simulink model "esempio_tutto"  (R2020b)
settings: Solver=VariableStepAuto  StartTime=0.0  StopTime=10.0  RelTol=1e-3
values from neighbouring files (symbols this model uses):
  b = [0,0,0]    [main_att.m]
  C_Kd = 5    [main_att.m]
  C_Kp = 5    [main_att.m]
  D = diag([0.5 1/3 0.25])    [main_att.m]
  j0 = diag([0.0109 0.0506 0.0509])    [main_att.m]
  jc = diag([0.00109 0.00109 0.00109])    [main_att.m]
  Kx = 0.012    [main_att.m]
  Ky = 0.01    [main_att.m]
  Kz = 0.008    [main_att.m]
  ng = [0.001,0.001,0.001]    [main_att.m]
  om_0 = 0.001    [main_att.m]
  R_Ka = 0.001    [main_att.m]
  R_Kd = 0.001    [main_att.m]
  R_Kl = 0.001    [main_att.m]
  R_Kn = 0.001    [main_att.m]
libraries: simulink_extras x3, vrlib x2
settings Model: Creator=jason  LastModifiedBy=jason

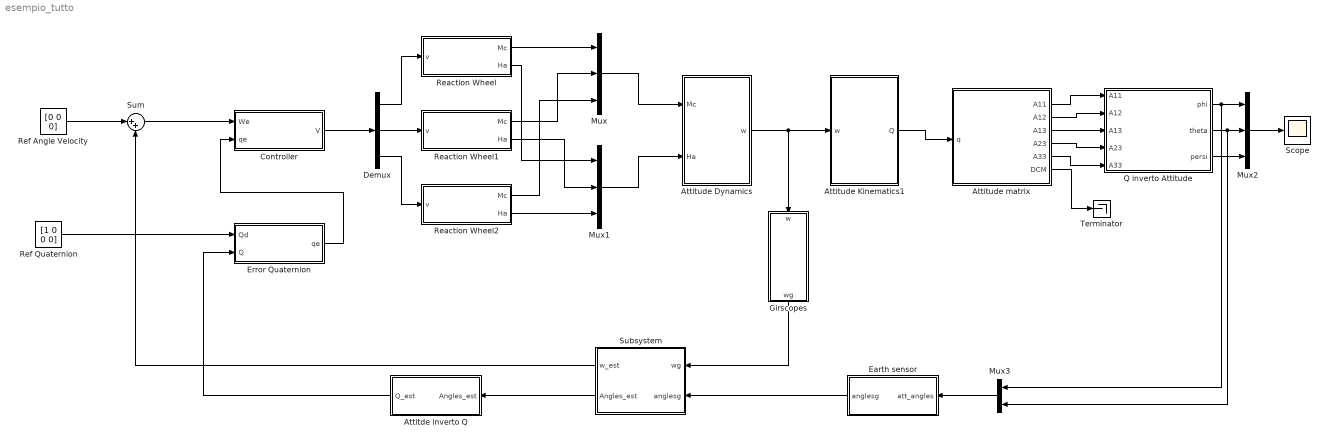
== system esempio_tutto ==
  Attitde inverto Q : Subsystem
  Attitude Dynamics : Subsystem
  Attitude Kinematics1 : Subsystem
  Attitude matrix : Subsystem
  Controller : Subsystem
  Demux : Demux  Outputs=3
  Earth sensor : Subsystem
  Error Quaternion : Subsystem
  Girscopes : Subsystem
  Mux : Mux  Inputs=3
  Mux1 : Mux  Inputs=3
  Mux2 : Mux  Inputs=3
  Mux3 : Mux  Inputs=2
  Q inverto Attitude : Subsystem
  Reaction Wheel : Subsystem
  Reaction Wheel1 : Subsystem
  Reaction Wheel2 : Subsystem
  Ref Angle Velocity : Constant  Value=[0 0 0]
  Ref Quaternion : Constant  Value=[1 0 0 0]
  Scope : Scope
  Subsystem : Subsystem
  Sum : Sum  Inputs=|++
  Terminator : Terminator
  wires:
  Sum/1 -> Controller/1(We)
  Ref Angle Velocity/1 -> Sum/1
  Error Quaternion/1(qe) -> Controller/2(qe)
  Ref Quaternion/1 -> Error Quaternion/1(Qd)
  Controller/1(V) -> Demux/1
  Demux/3 -> Reaction Wheel2/1(v)
  Demux/2 -> Reaction Wheel1/1(v)
  Demux/1 -> Reaction Wheel/1(v)
  Reaction Wheel/1(Mc) -> Mux/1
  Reaction Wheel1/1(Mc) -> Mux/2
  Reaction Wheel2/1(Mc) -> Mux/3
  Reaction Wheel/2(Ha) -> Mux1/1
  Reaction Wheel1/2(Ha) -> Mux1/2
  Reaction Wheel2/2(Ha) -> Mux1/3
  Mux/1 -> Attitude Dynamics/1(Mc)
  Mux1/1 -> Attitude Dynamics/2(Ha)
  Attitude Dynamics/1(w) -> Attitude Kinematics1/1(w), Girscopes/1(w)
  Attitude Kinematics1/1(Q) -> Attitude matrix/1(q)
  Attitude matrix/1(A11) -> Q inverto Attitude/1(A11)
  Attitude matrix/2(A12) -> Q inverto Attitude/2(A12)
  Attitude matrix/3(A13) -> Q inverto Attitude/3(A13)
  Attitude matrix/4(A23) -> Q inverto Attitude/4(A23)
  Attitude matrix/5(A33) -> Q inverto Attitude/5(A33)
  Q inverto Attitude/1(phi) -> Mux3/1, Mux2/1
  Q inverto Attitude/2(theta) -> Mux3/2, Mux2/2
  Q inverto Attitude/3(persi) -> Mux2/3
  Mux2/1 -> Scope/1
  Mux3/1 -> Earth sensor/1(att_angles)
  Girscopes/1(wg) -> Subsystem/1(wg)
  Earth sensor/1(anglesg) -> Subsystem/2(anglesg)
  Attitde inverto Q/1(Q_est) -> Error Quaternion/2(Q)
  Subsystem/2(Angles_est) -> Attitde inverto Q/1(Angles_est)
  Subsystem/1(w_est) -> Sum/2
  Attitude matrix/6(DCM) -> Terminator/1

== system esempio_tutto/Attitde inverto Q ==
  Angles_est : Inport
  MATLAB Function : MATLAB Function  TreatAsAtomicUnit=on
  Q_est : Outport
  wires:
  Angles_est/1 -> MATLAB Function/1(u)
  MATLAB Function/1(y) -> Q_est/1

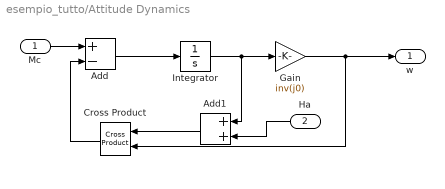
== system esempio_tutto/Attitude Dynamics ==
  Mc : Inport
  Ha : Inport  Port=2
  Add : Sum  Inputs=+-
  Add1 : Sum
  Cross Product : vrlib/Utilities/Cross Product
  Gain : Gain  Gain=inv(j0)
  Integrator : Integrator  InitialCondition=[0 0 0]
  w : Outport
  wires:
  Mc/1 -> Add/1
  Add/1 -> Integrator/1
  Integrator/1 -> Add1/1, Gain/1
  Gain/1 -> Cross Product/2, w/1
  Ha/1 -> Add1/2
  Add1/1 -> Cross Product/1
  Cross Product/1 -> Add/2

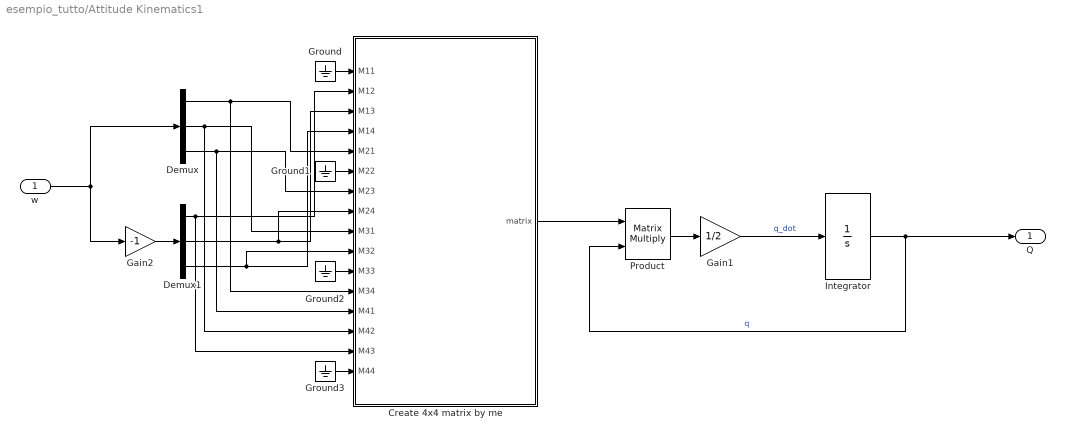
== system esempio_tutto/Attitude Kinematics1 ==
  w : Inport
  Create 4x4 matrix by me : Subsystem
  Demux : Demux  Outputs=3
  Demux1 : Demux  Outputs=3
  Gain1 : Gain  Gain=1/2
  Gain2 : Gain  Gain=-1
  Ground{,1..3} (4 alike) : Ground
  Integrator : Integrator  InitialCondition=[1 0 0 0]'
  Product : Product  Multiplication=Matrix(*)
  Q : Outport
  wires:
  Gain2/1 -> Demux1/1
  Demux/1 -> Create 4x4 matrix by me/12(M34), Create 4x4 matrix by me/5(M21)
  Demux/2 -> Create 4x4 matrix by me/14(M42), Create 4x4 matrix by me/9(M31)
  Demux/3 -> Create 4x4 matrix by me/13(M41), Create 4x4 matrix by me/7(M23)
  Demux1/1 -> Create 4x4 matrix by me/15(M43), Create 4x4 matrix by me/2(M12)
  Demux1/3 -> Create 4x4 matrix by me/10(M32), Create 4x4 matrix by me/4(M14)
  Demux1/2 -> Create 4x4 matrix by me/8(M24), Create 4x4 matrix by me/3(M13)
  Ground1/1 -> Create 4x4 matrix by me/6(M22)
  Ground/1 -> Create 4x4 matrix by me/1(M11)
  Ground2/1 -> Create 4x4 matrix by me/11(M33)
  Product/1 -> Gain1/1
  w/1 -> Demux/1, Gain2/1
  Gain1/1 -> Integrator/1  "q_dot"
  Ground3/1 -> Create 4x4 matrix by me/16(M44)
  Create 4x4 matrix by me/1(matrix) -> Product/1
  Integrator/1 -> Q/1, Product/2  "q"

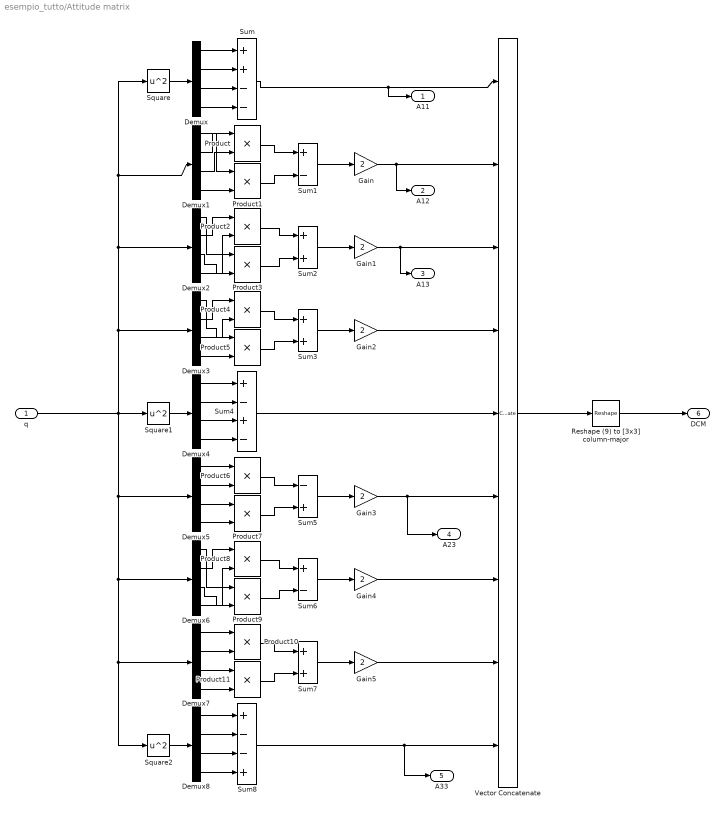
== system esempio_tutto/Attitude matrix ==
  q : Inport
  Demux{,1..8} (9 alike) : Demux
  Gain{,1..5} (6 alike) : Gain  Gain=2
  Product{,1..11} (12 alike) : Product
  Reshape (9) to [3x3] column-major : Reshape  OutputDimensionality=Customize  OutputDimensions=[3,3]
  Square : Math  Operator=square  SaturateOnIntegerOverflow=on
  Square1 : Math  Operator=square  SaturateOnIntegerOverflow=on
  Square2 : Math  Operator=square  SaturateOnIntegerOverflow=on
  Sum : Sum  Inputs=++--
  Sum1 : Sum  Inputs=+-
  Sum2 : Sum
  Sum3 : Sum
  Sum4 : Sum  Inputs=+-+-
  Sum5 : Sum  Inputs=-+
  Sum6 : Sum  Inputs=+-
  Sum7 : Sum
  Sum8 : Sum  Inputs=+--+
  Vector Concatenate : Concatenate  NumInputs=9
  A11 : Outport
  A12 : Outport  Port=2
  A13 : Outport  Port=3
  A23 : Outport  Port=4
  A33 : Outport  Port=5
  DCM : Outport  Port=6
  wires:
  Product10/1 -> Sum7/1
  Demux7/1 -> Product10/1
  Sum4/1 -> Vector Concatenate/5
  Product3/1 -> Sum2/2
  Demux5/4 -> Product7/2
  Gain5/1 -> Vector Concatenate/8
  Product11/1 -> Sum7/2
  Sum7/1 -> Gain5/1
  Gain4/1 -> Vector Concatenate/7
  Sum6/1 -> Gain4/1
  Demux5/2 -> Product6/2
  Demux7/2 -> Product10/2
  Demux5/3 -> Product7/1
  Demux5/1 -> Product6/1
  Product6/1 -> Sum5/1
  Demux3/1 -> Product5/1
  Demux6/4 -> Product8/2
  Sum3/1 -> Gain2/1
  Demux/1 -> Sum/1
  Demux6/1 -> Product9/1
  Demux4/3 -> Sum4/3
  Sum1/1 -> Gain/1
  Demux7/3 -> Product11/1
  Product7/1 -> Sum5/2
  Demux3/3 -> Product4/2
  Product4/1 -> Sum3/1
  Gain2/1 -> Vector Concatenate/4
  Demux1/3 -> Product/2
  Demux4/4 -> Sum4/4
  Demux2/2 -> Product2/1
  Product9/1 -> Sum6/2
  Demux2/1 -> Product3/1
  Demux2/4 -> Product2/2
  Demux4/2 -> Sum4/2
  Product1/1 -> Sum1/2
  Sum5/1 -> Gain3/1
  q/1 -> Square/1, Demux1/1, Demux2/1, Demux3/1, Square1/1, Demux5/1, Demux6/1, Demux7/1, Square2/1
  Product/1 -> Sum1/1
  Gain/1 -> A12/1, Vector Concatenate/2
  Product2/1 -> Sum2/1
  Sum2/1 -> Gain1/1
  Square/1 -> Demux/1
  Sum/1 -> A11/1, Vector Concatenate/1
  Demux/4 -> Sum/4
  Demux/2 -> Sum/2
  Demux3/2 -> Product4/1
  Demux6/2 -> Product8/1
  Demux/3 -> Sum/3
  Vector Concatenate/1 -> Reshape (9) to [3x3] column-major/1
  Product8/1 -> Sum6/1
  Demux8/4 -> Sum8/4
  Demux3/4 -> Product5/2
  Gain3/1 -> A23/1, Vector Concatenate/6
  Demux1/4 -> Product1/2
  Demux1/2 -> Product/1
  Demux7/4 -> Product11/2
  Demux8/2 -> Sum8/2
  Reshape (9) to [3x3] column-major/1 -> DCM/1
  Demux1/1 -> Product1/1
  Square2/1 -> Demux8/1
  Product5/1 -> Sum3/2
  Demux8/1 -> Sum8/1
  Square1/1 -> Demux4/1
  Sum8/1 -> A33/1, Vector Concatenate/9
  Gain1/1 -> A13/1, Vector Concatenate/3
  Demux4/1 -> Sum4/1
  Demux2/3 -> Product3/2
  Demux8/3 -> Sum8/3
  Demux6/3 -> Product9/2

== system esempio_tutto/Controller ==
  We : Inport
  qe : Inport  Port=2
  Gain : Gain  Gain=C_Kd  Multiplication=Matrix(K*u)
  Gain1 : Gain  Gain=C_Kp  Multiplication=Matrix(K*u)
  Quantizer : Quantizer
  Sum : Sum  Inputs=--
  V : Outport
  wires:
  We/1 -> Gain/1
  qe/1 -> Gain1/1
  Gain/1 -> Sum/1
  Gain1/1 -> Sum/2
  Sum/1 -> Quantizer/1
  Quantizer/1 -> V/1

== system esempio_tutto/Earth sensor ==
  att_angles : Inport
  Add : Sum  Inputs=+++
  Gain : Gain  Gain=b
  Quantizer : Quantizer
  Random Number : RandomNumber  Mean=0.01  SampleTime=0.1
  devi : Constant
  anglesg : Outport
  wires:
  att_angles/1 -> Add/1
  Add/1 -> Quantizer/1
  Quantizer/1 -> anglesg/1
  Random Number/1 -> Gain/1
  Gain/1 -> Add/3
  devi/1 -> Add/2

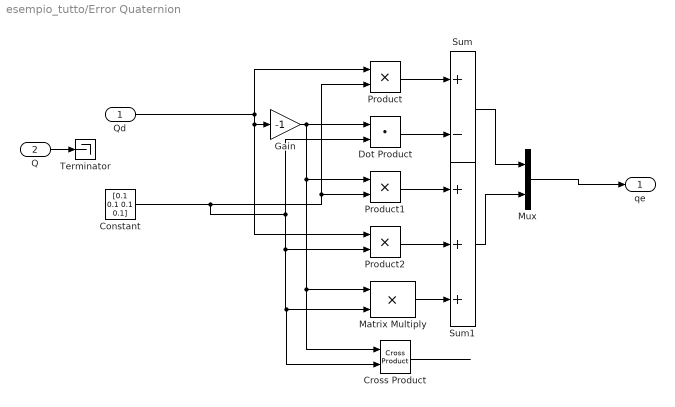
== system esempio_tutto/Error Quaternion ==
  Qd : Inport
  Q : Inport  Port=2
  Constant : Constant  Value=[0.1 0.1 0.1 0.1]
  Cross Product : vrlib/Utilities/Cross Product
  Dot Product : DotProduct  InputSameDT=on  OutDataTypeStr=Inherit: Inherit via internal rule
  Gain : Gain  Gain=-1
  Matrix Multiply : Product
  Mux : Mux  Inputs=2
  Product : Product
  Product1 : Product
  Product2 : Product
  Sum : Sum  Inputs=+-
  Sum1 : Sum  Inputs=+++
  Terminator : Terminator
  qe : Outport
  wires:
  Qd/1 -> Gain/1, Product2/1, Product/1
  Gain/1 -> Cross Product/1, Matrix Multiply/1, Product1/1, Dot Product/1
  Constant/1 -> Product/2, Product1/2, Cross Product/2, Matrix Multiply/2, Product2/2, Dot Product/2
  Product1/1 -> Sum1/1
  Product2/1 -> Sum1/2
  Matrix Multiply/1 -> Sum1/3
  Dot Product/1 -> Sum/2
  Product/1 -> Sum/1
  Sum/1 -> Mux/1
  Sum1/1 -> Mux/2
  Mux/1 -> qe/1
  Q/1 -> Terminator/1
  Cross Product/1 -> ?

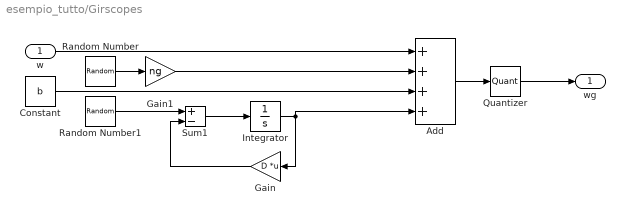
== system esempio_tutto/Girscopes ==
  w : Inport
  Add : Sum  Inputs=++++
  Constant : Constant  Value=b
  Gain : Gain  Gain=D  Multiplication=Matrix(K*u) (u vector)
  Gain1 : Gain  Gain=ng
  Integrator : Integrator  InitialCondition=nd'
  Quantizer : Quantizer
  Random Number : RandomNumber  SampleTime=0.1
  Random Number1 : RandomNumber  SampleTime=0.1
  Sum1 : Sum  Inputs=+-
  wg : Outport
  wires:
  Add/1 -> Quantizer/1
  Quantizer/1 -> wg/1
  w/1 -> Add/1
  Constant/1 -> Add/3
  Random Number/1 -> Gain1/1
  Gain1/1 -> Add/2
  Random Number1/1 -> Sum1/1
  Sum1/1 -> Integrator/1
  Integrator/1 -> Gain/1, Add/4
  Gain/1 -> Sum1/2

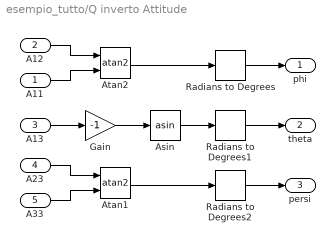
== system esempio_tutto/Q inverto Attitude ==
  A11 : Inport
  A12 : Inport  Port=2
  A13 : Inport  Port=3
  A23 : Inport  Port=4
  A33 : Inport  Port=5
  Asin : Trigonometry  Operator=asin
  Atan1 : Trigonometry  Operator=atan2
  Atan2 : Trigonometry  Operator=atan2
  Gain : Gain  Gain=-1
  Radians to Degrees : simulink_extras/Transformations/Radians to Degrees
  Radians to Degrees1 : simulink_extras/Transformations/Radians to Degrees
  Radians to Degrees2 : simulink_extras/Transformations/Radians to Degrees
  phi : Outport
  theta : Outport  Port=2
  persi : Outport  Port=3
  wires:
  A11/1 -> Atan2/2
  A12/1 -> Atan2/1
  A23/1 -> Atan1/1
  A33/1 -> Atan1/2
  A13/1 -> Gain/1
  Gain/1 -> Asin/1
  Atan2/1 -> Radians to Degrees/1
  Asin/1 -> Radians to Degrees1/1
  Atan1/1 -> Radians to Degrees2/1
  Radians to Degrees/1 -> phi/1
  Radians to Degrees1/1 -> theta/1
  Radians to Degrees2/1 -> persi/1

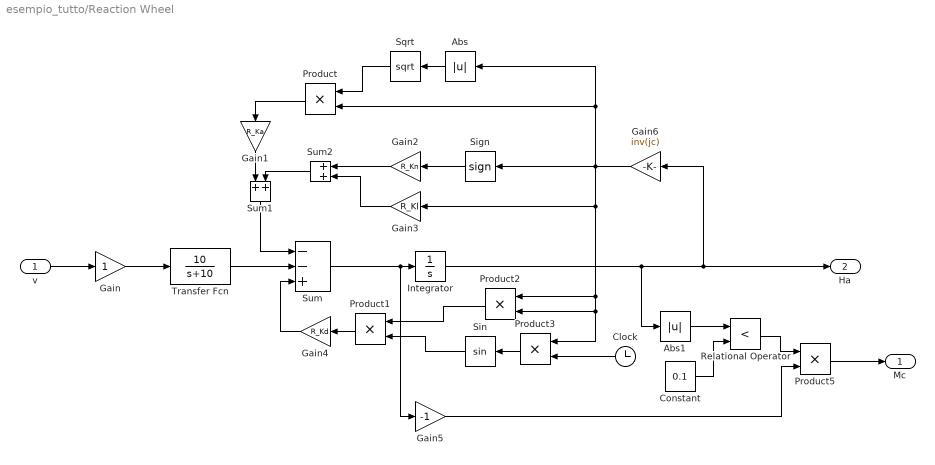
== system esempio_tutto/Reaction Wheel ==
  v : Inport
  Abs : Abs
  Abs1 : Abs
  Clock : Clock
  Constant : Constant  Value=0.1
  Gain : Gain
  Gain1 : Gain  Gain=R_Ka
  Gain2 : Gain  Gain=R_Kn
  Gain3 : Gain  Gain=R_Kl
  Gain4 : Gain  Gain=R_Kd
  Gain5 : Gain  Gain=-1
  Gain6 : Gain  Gain=inv(jc)
  Integrator : Integrator
  Product{,1..3,5} (5 alike) : Product
  Relational Operator : RelationalOperator  Operator=<  OutDataTypeStr=boolean  RndMeth=Simplest
  Sign : Signum
  Sin : Trigonometry
  Sqrt : Sqrt  SaturateOnIntegerOverflow=on
  Sum : Sum  Inputs=--+
  Sum1 : Sum
  Sum2 : Sum
  Transfer Fcn : TransferFcn  Numerator=[10]  Denominator=[1 10]
  Mc : Outport
  Ha : Outport  Port=2
  wires:
  Gain/1 -> Transfer Fcn/1
  Transfer Fcn/1 -> Sum/2
  Sum1/1 -> Sum/1
  Sum2/1 -> Sum1/2
  Gain1/1 -> Sum1/1
  Product/1 -> Gain1/1
  Abs/1 -> Sqrt/1
  Sqrt/1 -> Product/1
  Gain2/1 -> Sum2/1
  Sign/1 -> Gain2/1
  Gain3/1 -> Sum2/2
  Gain4/1 -> Sum/3
  Product1/1 -> Gain4/1
  Product3/1 -> Sin/1
  Sin/1 -> Product1/2
  Sum/1 -> Gain5/1, Integrator/1
  Integrator/1 -> Abs1/1, Ha/1, Gain6/1
  Gain6/1 -> Gain3/1, Product2/1, Product3/1, Product2/2, Product/2, Abs/1, Sign/1
  Clock/1 -> Product3/2
  Abs1/1 -> Relational Operator/1
  Constant/1 -> Relational Operator/2
  Relational Operator/1 -> Product5/1
  Gain5/1 -> Product5/2
  Product5/1 -> Mc/1
  Product2/1 -> Product1/1
  v/1 -> Gain/1

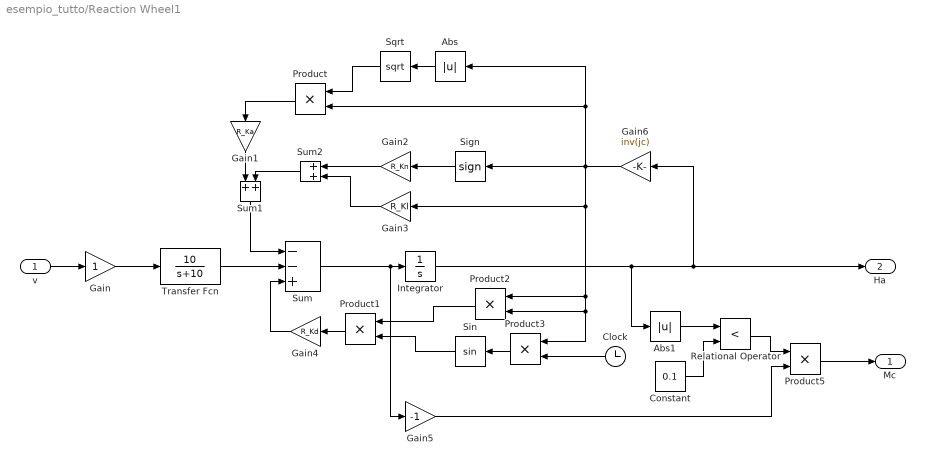
== system esempio_tutto/Reaction Wheel1 ==
  v : Inport
  Abs : Abs
  Abs1 : Abs
  Clock : Clock
  Constant : Constant  Value=0.1
  Gain : Gain
  Gain1 : Gain  Gain=R_Ka
  Gain2 : Gain  Gain=R_Kn
  Gain3 : Gain  Gain=R_Kl
  Gain4 : Gain  Gain=R_Kd
  Gain5 : Gain  Gain=-1
  Gain6 : Gain  Gain=inv(jc)
  Integrator : Integrator
  Product{,1..3,5} (5 alike) : Product
  Relational Operator : RelationalOperator  Operator=<  OutDataTypeStr=boolean  RndMeth=Simplest
  Sign : Signum
  Sin : Trigonometry
  Sqrt : Sqrt  SaturateOnIntegerOverflow=on
  Sum : Sum  Inputs=--+
  Sum1 : Sum
  Sum2 : Sum
  Transfer Fcn : TransferFcn  Numerator=[10]  Denominator=[1 10]
  Mc : Outport
  Ha : Outport  Port=2
  wires:
  Sum1/1 -> Sum/1
  Product3/1 -> Sin/1
  Relational Operator/1 -> Product5/1
  Sum/1 -> Gain5/1, Integrator/1
  Constant/1 -> Relational Operator/2
  Abs1/1 -> Relational Operator/1
  Clock/1 -> Product3/2
  Product2/1 -> Product1/1
  Transfer Fcn/1 -> Sum/2
  Product1/1 -> Gain4/1
  Gain5/1 -> Product5/2
  Gain1/1 -> Sum1/1
  Sin/1 -> Product1/2
  Integrator/1 -> Abs1/1, Ha/1, Gain6/1
  Gain3/1 -> Sum2/2
  Sum2/1 -> Sum1/2
  Product5/1 -> Mc/1
  Gain4/1 -> Sum/3
  Gain6/1 -> Gain3/1, Product2/1, Product3/1, Product2/2, Product/2, Abs/1, Sign/1
  Sign/1 -> Gain2/1
  Gain2/1 -> Sum2/1
  Sqrt/1 -> Product/1
  Product/1 -> Gain1/1
  Abs/1 -> Sqrt/1
  Gain/1 -> Transfer Fcn/1
  v/1 -> Gain/1

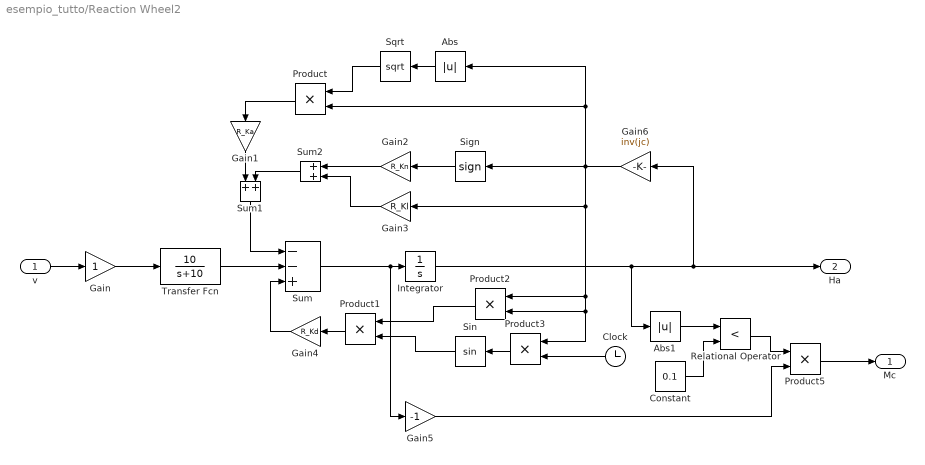
== system esempio_tutto/Reaction Wheel2 ==
  v : Inport
  Abs : Abs
  Abs1 : Abs
  Clock : Clock
  Constant : Constant  Value=0.1
  Gain : Gain
  Gain1 : Gain  Gain=R_Ka
  Gain2 : Gain  Gain=R_Kn
  Gain3 : Gain  Gain=R_Kl
  Gain4 : Gain  Gain=R_Kd
  Gain5 : Gain  Gain=-1
  Gain6 : Gain  Gain=inv(jc)
  Integrator : Integrator
  Product{,1..3,5} (5 alike) : Product
  Relational Operator : RelationalOperator  Operator=<  OutDataTypeStr=boolean  RndMeth=Simplest
  Sign : Signum
  Sin : Trigonometry
  Sqrt : Sqrt  SaturateOnIntegerOverflow=on
  Sum : Sum  Inputs=--+
  Sum1 : Sum
  Sum2 : Sum
  Transfer Fcn : TransferFcn  Numerator=[10]  Denominator=[1 10]
  Mc : Outport
  Ha : Outport  Port=2
  wires:
  Sum1/1 -> Sum/1
  Product3/1 -> Sin/1
  Relational Operator/1 -> Product5/1
  Sum/1 -> Gain5/1, Integrator/1
  Constant/1 -> Relational Operator/2
  Abs1/1 -> Relational Operator/1
  Clock/1 -> Product3/2
  Product2/1 -> Product1/1
  Transfer Fcn/1 -> Sum/2
  Product1/1 -> Gain4/1
  Gain5/1 -> Product5/2
  Gain1/1 -> Sum1/1
  Sin/1 -> Product1/2
  Integrator/1 -> Abs1/1, Ha/1, Gain6/1
  Gain3/1 -> Sum2/2
  Sum2/1 -> Sum1/2
  Product5/1 -> Mc/1
  Gain4/1 -> Sum/3
  v/1 -> Gain/1
  Gain6/1 -> Gain3/1, Product2/1, Product3/1, Product2/2, Product/2, Abs/1, Sign/1
  Sign/1 -> Gain2/1
  Gain2/1 -> Sum2/1
  Sqrt/1 -> Product/1
  Product/1 -> Gain1/1
  Abs/1 -> Sqrt/1
  Gain/1 -> Transfer Fcn/1

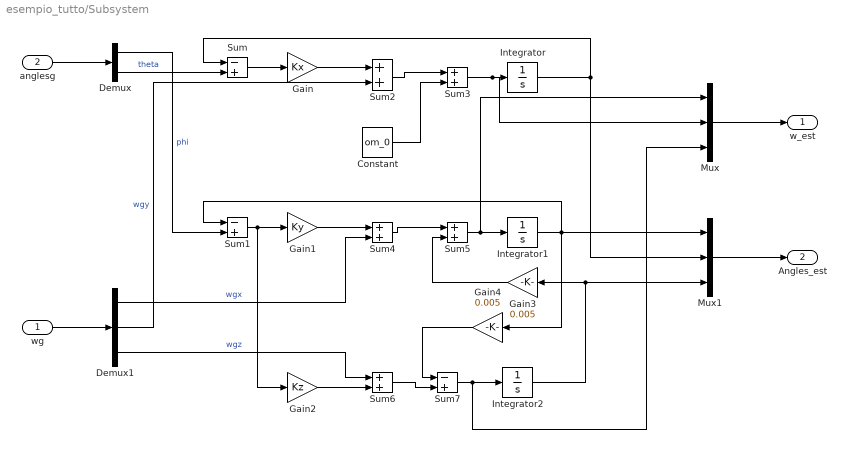
== system esempio_tutto/Subsystem ==
  wg : Inport
  anglesg : Inport  Port=2
  Constant : Constant  Value=om_0
  Demux : Demux  Outputs=2
  Demux1 : Demux  Outputs=3
  Gain : Gain  Gain=Kx
  Gain1 : Gain  Gain=Ky
  Gain2 : Gain  Gain=Kz
  Gain3 : Gain  Gain=0.005
  Gain4 : Gain  Gain=0.005
  Integrator : Integrator
  Integrator1 : Integrator
  Integrator2 : Integrator
  Mux : Mux  Inputs=3
  Mux1 : Mux  Inputs=3
  Sum : Sum  Inputs=-+
  Sum1 : Sum  Inputs=-+
  Sum{2..6} (5 alike) : Sum
  Sum7 : Sum  Inputs=-+
  w_est : Outport
  Angles_est : Outport  Port=2
  wires:
  anglesg/1 -> Demux/1
  wg/1 -> Demux1/1
  Demux/2 -> Sum/2  "theta"
  Demux/1 -> Sum1/2  "phi"
  Sum/1 -> Gain/1
  Sum1/1 -> Gain2/1, Gain1/1
  Gain/1 -> Sum2/1
  Sum2/1 -> Sum3/1
  Sum3/1 -> Mux/2, Integrator/1
  Constant/1 -> Sum3/2
  Demux1/2 -> Sum2/2  "wgy"
  Gain1/1 -> Sum4/1
  Sum4/1 -> Sum5/1
  Sum5/1 -> Integrator1/1, Mux/1
  Gain2/1 -> Sum6/2
  Sum6/1 -> Sum7/2
  Demux1/3 -> Sum6/1  "wgz"
  Demux1/1 -> Sum4/2  "wgx"
  Integrator1/1 -> Gain4/1, Mux1/1, Sum1/1
  Gain3/1 -> Sum5/2
  Sum7/1 -> Mux/3, Integrator2/1
  Gain4/1 -> Sum7/1
  Integrator2/1 -> Gain3/1, Mux1/3
  Integrator/1 -> Mux1/2, Sum/1
  Mux1/1 -> Angles_est/1
  Mux/1 -> w_est/1

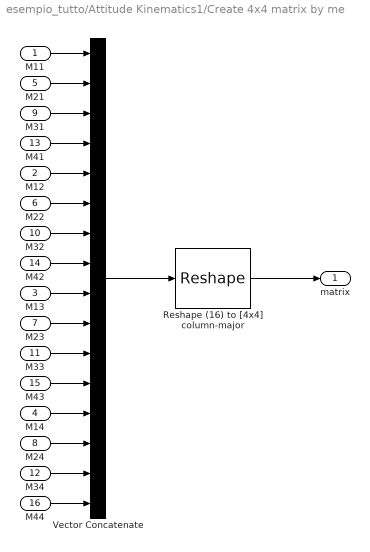
== system esempio_tutto/Attitude Kinematics1/Create 4x4 matrix by me ==
  M11 : Inport
  M12 : Inport  Port=2
  M13 : Inport  Port=3
  M14 : Inport  Port=4
  M21 : Inport  Port=5
  M22 : Inport  Port=6
  M23 : Inport  Port=7
  M24 : Inport  Port=8
  M31 : Inport  Port=9
  M32 : Inport  Port=10
  M33 : Inport  Port=11
  M34 : Inport  Port=12
  M41 : Inport  Port=13
  M42 : Inport  Port=14
  M43 : Inport  Port=15
  M44 : Inport  Port=16
  Reshape (16) to [4x4] column-major : Reshape  OutputDimensionality=Customize  OutputDimensions=[4,4]
  Vector Concatenate : Concatenate  NumInputs=16
  matrix : Outport
  wires:
  M12/1 -> Vector Concatenate/5
  M11/1 -> Vector Concatenate/1
  M13/1 -> Vector Concatenate/9
  M14/1 -> Vector Concatenate/13
  M21/1 -> Vector Concatenate/2
  M44/1 -> Vector Concatenate/16
  M34/1 -> Vector Concatenate/15
  M24/1 -> Vector Concatenate/14
  M43/1 -> Vector Concatenate/12
  M33/1 -> Vector Concatenate/11
  M23/1 -> Vector Concatenate/10
  M42/1 -> Vector Concatenate/8
  M32/1 -> Vector Concatenate/7
  M22/1 -> Vector Concatenate/6
  M41/1 -> Vector Concatenate/4
  M31/1 -> Vector Concatenate/3
  Vector Concatenate/1 -> Reshape (16) to [4x4] column-major/1
  Reshape (16) to [4x4] column-major/1 -> matrix/1

== matlab function esempio_tutto/Attitde inverto Q/MATLAB Function ==
  data: u input; y output
function y = fcn(u)
a = cos(u(1)/2)*cos(u(2)/2)*cos(u(3)/2) +sin(u(1)/2)*sin(u(2)/2)*sin(u(3)/2);
b = sin(u(1)/2)*cos(u(2)/2)*cos(u(3)/2) -cos(u(1)/2)*sin(u(2)/2)*sin(u(3)/2);
c = cos(u(1)/2)*sin(u(2)/2)*cos(u(3)/2) +sin(u(1)/2)*cos(u(2)/2)*sin(u(3)/2);
d = cos(u(1)/2)*cos(u(2)/2)*sin(u(3)/2) +sin(u(1)/2)*sin(u(2)/2)*cos(u(3)/2);
y = [a b c d];
end
